simulink model "Motor_Dynamics_practice1_2025a"  (R2025a)
settings: Solver=VariableStepAuto  StartTime=0.0  StopTime=10.0  RelTol=1e-3
InitFcn:
  | %% Motor parameter
  | 
  | rad2rpm = 60 / (2 * pi);
  | 
  | rpm2rad = 1 / rad2rpm;
  | 
  | Friction_Coef = 0.0001;         %[N m /s]
  | 
  | Inertia = 2.8e-05;              %[kg m^2]
  | 
  | Resistance = 0.1170;            %[ohm]
  | 
  | K_Torque = 1 / (rpm2rad * 960); %[N m/A]
  | 
  | K_Emf = K_Torque;                 %[V s/rad]
settings Model: Creator=user  LastModifiedBy=user

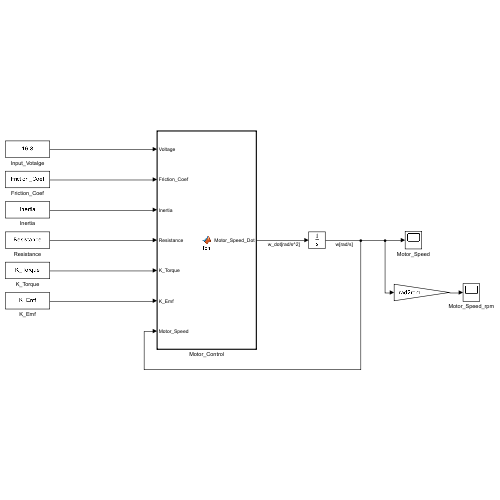
[thumbnail: Simulink's stored preview of the top-level diagram]
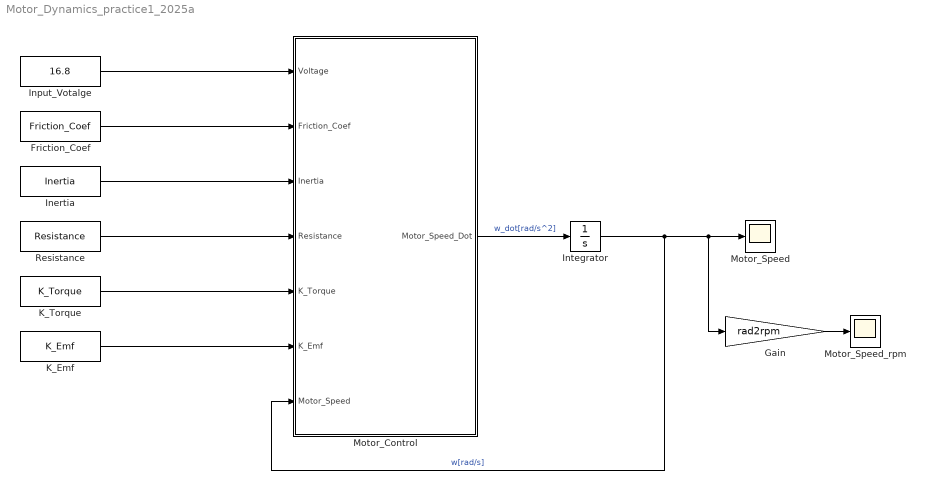
== system Motor_Dynamics_practice1_2025a ==
  Friction_Coef : Constant  Value=Friction_Coef
  Gain : Gain  Gain=rad2rpm
  Inertia : Constant  Value=Inertia
  Input_Votalge : Constant  Value=16.8
  Integrator : Integrator
  K_Emf : Constant  Value=K_Emf
  K_Torque : Constant  Value=K_Torque
  Motor_Control : MATLAB Function  TreatAsAtomicUnit=on
  Motor_Speed : Scope
      settings: Title=Lec1  ActiveDisplayYMinimum=-188.77633392926  ActiveDisplayYMaximum=1698.9870053633404  YLabel=rad/s
  Motor_Speed_rpm : Scope
      settings: Title=Lec1  ActiveDisplayYMinimum=-1802.6812010164804  ActiveDisplayYMaximum=16224.130809148328  YLabel=rpm
  Resistance : Constant  Value=Resistance
  wires:
  Integrator/1 -> Gain/1, Motor_Speed/1, Motor_Control/7(Motor_Speed)  "w[rad/s]"
  Motor_Control/1(Motor_Speed_Dot) -> Integrator/1  "w_dot[rad/s^2]"
  Gain/1 -> Motor_Speed_rpm/1
  Input_Votalge/1 -> Motor_Control/1(Voltage)
  Friction_Coef/1 -> Motor_Control/2(Friction_Coef)
  Inertia/1 -> Motor_Control/3(Inertia)
  Resistance/1 -> Motor_Control/4(Resistance)
  K_Torque/1 -> Motor_Control/5(K_Torque)
  K_Emf/1 -> Motor_Control/6(K_Emf)

== matlab function Motor_Dynamics_practice1_2025a/Motor_Control ==
  data: Voltage input; Friction_Coef input; Inertia input; Resistance input; K_Torque input; K_Emf input; Motor_Speed_Dot output; Motor_Speed input
function Motor_Speed_Dot = fcn(Voltage, Friction_Coef, Inertia, Resistance, K_Torque, K_Emf, Motor_Speed)

V_Emf = K_Emf * Motor_Speed; %[Voltage]

Current = (Voltage - V_Emf) / Resistance; %[A]

Motor_Speed_Dot = (K_Torque * Current - Friction_Coef * Motor_Speed)/ Inertia; %[rad/s^2]

end
